simulink model "LongitudinalControlDesignPitchRate"  (R2020b)
settings: Solver=ode15s  StartTime=0.0  StopTime=550  RelTol=1e-3
values from neighbouring files (symbols this model uses):
  actuatorDen = [1,   actuatorTimeConstant]    [LateralControl.m]    (also in LongitudinalControl.m)
  actuatorNum = actuatorGain*actuatorTimeConstant    (= 5)    [LateralControl.m]    (also in LongitudinalControl.m)
  ALong = [	-0.0141295      0.0580298       0           -9.81 ... (first row only)    [LongitudinalControl.m]
  AShortPeriod = ALong(2:3,2:3)    [LongitudinalControl.m]
  BLong = [	-0.1703679 ... (first row only)    [LongitudinalControl.m]
  BShortPeriod = BLong(2:3)    [LongitudinalControl.m]
  CLong = [1,     0,  0,  0 ... (first row only)    [LongitudinalControl.m]
  CShortPeriod = CLong(2:3,2:3)    [LongitudinalControl.m]
  DGain = PGain*Td    (= 0.0211)    [LateralControl.m]    (also in LongitudinalControl.m)
  DLong = [0 ... (first row only)    [LongitudinalControl.m]
  DShortPeriod = DLong(2:3)    [LongitudinalControl.m]
  InitialConditions = [0 ... (first row only)    [LateralControl.m]    (also in LongitudinalControl.m)
  PGain = 0.211    [LateralControl.m]    (also in LongitudinalControl.m)
  stepCommand = 0    [LateralControl.m]    (also in LongitudinalControl.m = 1)
libraries: slpidlib x2
settings Model: Creator=Antonis Kantounias  LastModifiedBy=Antonis Kantounias

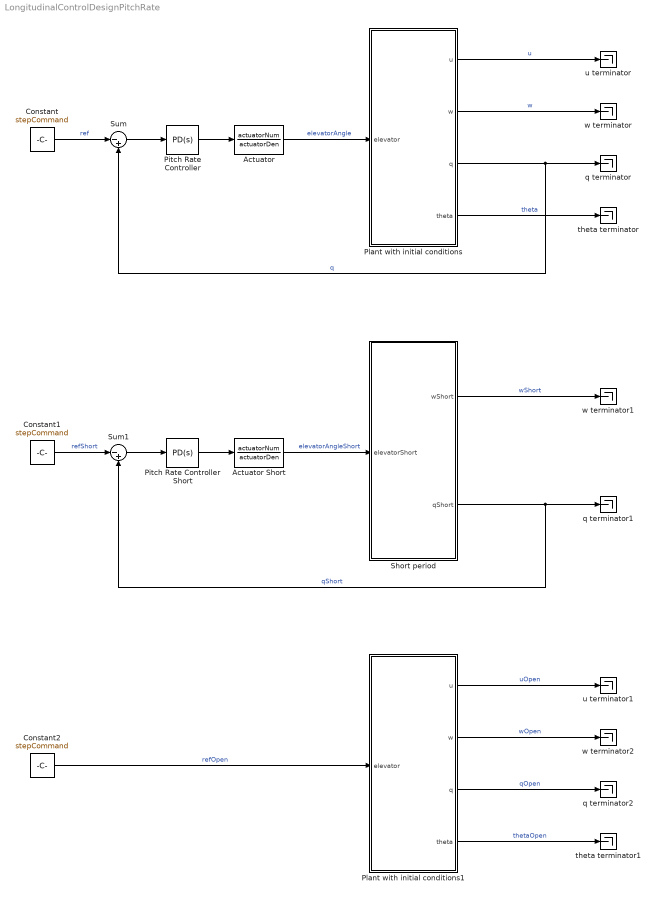
== system LongitudinalControlDesignPitchRate ==
  Actuator : TransferFcn  Numerator=actuatorNum  Denominator=actuatorDen
  Actuator Short : TransferFcn  Numerator=actuatorNum  Denominator=actuatorDen
  Constant : Constant  Value=stepCommand
  Constant1 : Constant  Value=stepCommand
  Constant2 : Constant  Value=stepCommand
  Pitch Rate Controller : slpidlib/PID Controller  Controller=PD  Form=Parallel  TimeDomain=Continuous-time  UseExternalTs=off  SampleTime=-1  IntegratorMethod=Forward Euler  FilterMethod=Forward Euler  ControllerParametersSource=internal  P=PGain  I=1  D=DGain  UseFilter=on  N=100  TunerSelectOption=Transfer Function Based (PID Tuner App)  InitialConditionSource=internal  InitialConditionForIntegrator=0  InitialConditionForFilter=0  DifferentiatorICPrevScaledInput=0  ExternalReset=none  TrackingMode=off  Kt=1  LimitOutput=off  SatLimitsSource=internal  UpperSaturationLimit=inf  LowerSaturationLimit=-inf  LinearizeAsGain=on  AntiWindupMode=none  Kb=1  POutMin=[]  POutMax=[]  IOutMin=[]  IOutMax=[]  DOutMin=[]  DOutMax=[]  NOutMin=[]  NOutMax=[]  SumOutMin=[]  SumOutMax=[]  SaturationOutMin=[]  SaturationOutMax=[]  PParamMin=[]  PParamMax=[]  IParamMin=[]  IParamMax=[]  DParamMin=[]  DParamMax=[]  NParamMin=[]  NParamMax=[]  KbParamMin=[]  KbParamMax=[]  KtParamMin=[]  KtParamMax=[]  KbOutMin=[]  KbOutMax=[]  KtOutMin=[]  KtOutMax=[]  IntegratorOutMin=[]  IntegratorOutMax=[]  FilterOutMin=[]  FilterOutMax=[]  SumI1OutMin=[]  SumI1OutMax=[]  SumI2OutMin=[]  SumI2OutMax=[]  SumI3OutMin=[]  SumI3OutMax=[]  SumI4OutMin=[]  SumI4OutMax=[]  SumDOutMin=[]  SumDOutMax=[]  DifferentiatorOutMin=[]  DifferentiatorOutMax=[]  FilterDiffOutCoefMin=[]  FilterDiffOutCoefMax=[]  ReciprocalOutMin=[]  ReciprocalOutMax=[]  SumDenOutMin=[]  SumDenOutMax=[]  SumNumOutMin=[]  SumNumOutMax=[]  DivideOutMin=[]  DivideOutMax=[]  UdiffTsProdOutMin=[]  UdiffTsProdOutMax=[]  NTsProdOutMin=[]  NTsProdOutMax=[]  UintegralTsProdOutMin=[]  UintegralTsProdOutMax=[]  UngainTsProdOutMin=[]  UngainTsProdOutMax=[]  IntegratorContinuousStateAttributes=''  IntegratorStateMustResolveToSignalObject=off  IntegratorRTWStateStorageClass=Auto  FilterContinuousStateAttributes=''  FilterStateMustResolveToSignalObject=off  FilterRTWStateStorageClass=Auto  ParallelPVariant=InternalParameters  IdealPVariant=Disabled  IVariant=Disabled  DVariant=InternalParameters  IntegratorVariant=Disabled  SatVariant=Disabled  AWVariant=Disabled  PCopyVariant=Disabled  TRVariant=Disabled  FdbkBlocksVariant=Forward  IdealPFdbkVariant=Disabled  SatFdbkVariant=Disabled  DerivativeFilterVariant=ContFilter  NVariant=InternalParameters  NCopyVariant=Disabled  FilterICVariant=InternalICsFilter  IntegratorICVariant=Disabled  ExternalResetVariant=Disabled  TRSumVariant=Passthrough  SumFdbkVariant=Disabled  SumVariant=Sum_PD  TsampFilterVariant=InternalTs  TsampNgainVariant=Passthrough  TsampIntegralVariant=Disabled_SignalSpec  ExternalSaturationOutDataTypeStr=Inherit: Same as second input
  Pitch Rate Controller Short : slpidlib/PID Controller  Controller=PD  Form=Parallel  TimeDomain=Continuous-time  UseExternalTs=off  SampleTime=-1  IntegratorMethod=Forward Euler  FilterMethod=Forward Euler  ControllerParametersSource=internal  P=PGain  I=1  D=DGain  UseFilter=on  N=100  TunerSelectOption=Transfer Function Based (PID Tuner App)  InitialConditionSource=internal  InitialConditionForIntegrator=0  InitialConditionForFilter=0  DifferentiatorICPrevScaledInput=0  ExternalReset=none  TrackingMode=off  Kt=1  LimitOutput=off  SatLimitsSource=internal  UpperSaturationLimit=inf  LowerSaturationLimit=-inf  LinearizeAsGain=on  AntiWindupMode=none  Kb=1  POutMin=[]  POutMax=[]  IOutMin=[]  IOutMax=[]  DOutMin=[]  DOutMax=[]  NOutMin=[]  NOutMax=[]  SumOutMin=[]  SumOutMax=[]  SaturationOutMin=[]  SaturationOutMax=[]  PParamMin=[]  PParamMax=[]  IParamMin=[]  IParamMax=[]  DParamMin=[]  DParamMax=[]  NParamMin=[]  NParamMax=[]  KbParamMin=[]  KbParamMax=[]  KtParamMin=[]  KtParamMax=[]  KbOutMin=[]  KbOutMax=[]  KtOutMin=[]  KtOutMax=[]  IntegratorOutMin=[]  IntegratorOutMax=[]  FilterOutMin=[]  FilterOutMax=[]  SumI1OutMin=[]  SumI1OutMax=[]  SumI2OutMin=[]  SumI2OutMax=[]  SumI3OutMin=[]  SumI3OutMax=[]  SumI4OutMin=[]  SumI4OutMax=[]  SumDOutMin=[]  SumDOutMax=[]  DifferentiatorOutMin=[]  DifferentiatorOutMax=[]  FilterDiffOutCoefMin=[]  FilterDiffOutCoefMax=[]  ReciprocalOutMin=[]  ReciprocalOutMax=[]  SumDenOutMin=[]  SumDenOutMax=[]  SumNumOutMin=[]  SumNumOutMax=[]  DivideOutMin=[]  DivideOutMax=[]  UdiffTsProdOutMin=[]  UdiffTsProdOutMax=[]  NTsProdOutMin=[]  NTsProdOutMax=[]  UintegralTsProdOutMin=[]  UintegralTsProdOutMax=[]  UngainTsProdOutMin=[]  UngainTsProdOutMax=[]  IntegratorContinuousStateAttributes=''  IntegratorStateMustResolveToSignalObject=off  IntegratorRTWStateStorageClass=Auto  FilterContinuousStateAttributes=''  FilterStateMustResolveToSignalObject=off  FilterRTWStateStorageClass=Auto  ParallelPVariant=InternalParameters  IdealPVariant=Disabled  IVariant=Disabled  DVariant=InternalParameters  IntegratorVariant=Disabled  SatVariant=Disabled  AWVariant=Disabled  PCopyVariant=Disabled  TRVariant=Disabled  FdbkBlocksVariant=Forward  IdealPFdbkVariant=Disabled  SatFdbkVariant=Disabled  DerivativeFilterVariant=ContFilter  NVariant=InternalParameters  NCopyVariant=Disabled  FilterICVariant=InternalICsFilter  IntegratorICVariant=Disabled  ExternalResetVariant=Disabled  TRSumVariant=Passthrough  SumFdbkVariant=Disabled  SumVariant=Sum_PD  TsampFilterVariant=InternalTs  TsampNgainVariant=Passthrough  TsampIntegralVariant=Disabled_SignalSpec  ExternalSaturationOutDataTypeStr=Inherit: Same as second input
  Plant with initial conditions : Subsystem
  Plant with initial conditions1 : Subsystem
  Short period : Subsystem
  Sum : Sum  Inputs=|-+
  Sum1 : Sum  Inputs=|-+
  q terminator : Terminator
  q terminator1 : Terminator
  q terminator2 : Terminator
  theta terminator : Terminator
  theta terminator1 : Terminator
  u terminator : Terminator
  u terminator1 : Terminator
  w terminator : Terminator
  w terminator1 : Terminator
  w terminator2 : Terminator
  wires:
  Plant with initial conditions/3(q) -> q terminator/1, Sum/2  "q"
  Plant with initial conditions/1(u) -> u terminator/1  "u"
  Plant with initial conditions/2(w) -> w terminator/1  "w"
  Plant with initial conditions/4(theta) -> theta terminator/1  "theta"
  Constant/1 -> Sum/1  "ref"
  Sum/1 -> Pitch Rate Controller/1
  Pitch Rate Controller/1 -> Actuator/1
  Actuator/1 -> Plant with initial conditions/1(elevator)  "elevatorAngle"
  Actuator Short/1 -> Short period/1(elevatorShort)  "elevatorAngleShort"
  Pitch Rate Controller Short/1 -> Actuator Short/1
  Sum1/1 -> Pitch Rate Controller Short/1
  Constant1/1 -> Sum1/1  "refShort"
  Short period/1(wShort) -> w terminator1/1  "wShort"
  Short period/2(qShort) -> Sum1/2, q terminator1/1  "qShort"
  Constant2/1 -> Plant with initial conditions1/1(elevator)  "refOpen"
  Plant with initial conditions1/4(theta) -> theta terminator1/1  "thetaOpen"
  Plant with initial conditions1/1(u) -> u terminator1/1  "uOpen"
  Plant with initial conditions1/2(w) -> w terminator2/1  "wOpen"
  Plant with initial conditions1/3(q) -> q terminator2/1  "qOpen"

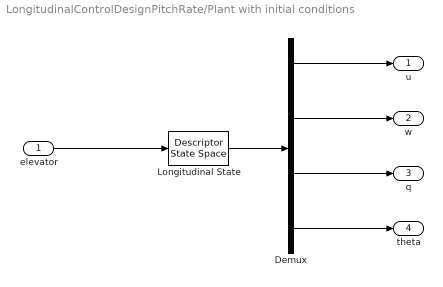
== system LongitudinalControlDesignPitchRate/Plant with initial conditions ==
  elevator : Inport
  Demux : Demux
  "Longitudinal State " : DescriptorStateSpace  E=ELong  A=ALong  B=BLong  C=CLong  D=DLong  InitialCondition=InitialConditions  ContinuousStateAttributes='LongitudinalSystem'
  u : Outport
  w : Outport  Port=2
  q : Outport  Port=3
  theta : Outport  Port=4
  wires:
  "Longitudinal State "/1 -> Demux/1
  Demux/4 -> theta/1
  Demux/1 -> u/1
  Demux/3 -> q/1
  Demux/2 -> w/1
  elevator/1 -> "Longitudinal State "/1

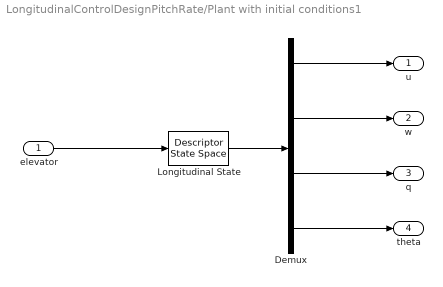
== system LongitudinalControlDesignPitchRate/Plant with initial conditions1 ==
  elevator : Inport
  Demux : Demux
  "Longitudinal State " : DescriptorStateSpace  E=ELong  A=ALong  B=BLong  C=CLong  D=DLong  InitialCondition=InitialConditions  ContinuousStateAttributes='LongitudinalSystem'
  u : Outport
  w : Outport  Port=2
  q : Outport  Port=3
  theta : Outport  Port=4
  wires:
  elevator/1 -> "Longitudinal State "/1
  Demux/2 -> w/1
  Demux/3 -> q/1
  Demux/1 -> u/1
  Demux/4 -> theta/1
  "Longitudinal State "/1 -> Demux/1

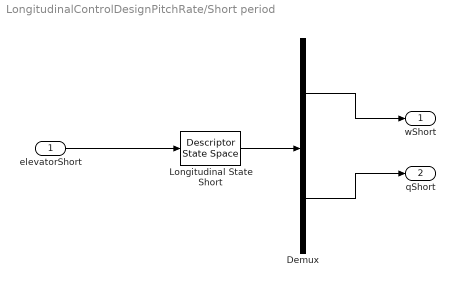
== system LongitudinalControlDesignPitchRate/Short period ==
  elevatorShort : Inport
  Demux : Demux  Outputs=2
  "Longitudinal State Short " : DescriptorStateSpace  E=[1,0;0,1]  A=AShortPeriod  B=BShortPeriod  C=CShortPeriod  D=DShortPeriod  InitialCondition=InitialConditions(2:3)  ContinuousStateAttributes='LongitudinalSystem'
  wShort : Outport
  qShort : Outport  Port=2
  wires:
  elevatorShort/1 -> "Longitudinal State Short "/1
  Demux/2 -> qShort/1
  "Longitudinal State Short "/1 -> Demux/1
  Demux/1 -> wShort/1
